simulink subsystem "RT_DynamicInflow_V1_2"  (R2025a)
settings: Solver=VariableStepAuto  StartTime=0.0  StopTime=100  RelTol=1e-3
model mask{RT_BEDistFromEffSta=0, RT_AirDensity=0, RT_RotorRadius=0}
  mask prompts: RT_BEDistFromEffSta "Blade element distance from effective station [-]"; RT_AirDensity "Air density [kgm^-3]"; RT_RotorRadius "Rotor radius [m]"
settings Model: DefaultTestHarness=RT_DynamicInflow_Harness1  Creator=Admin  LastModifiedBy=Admin

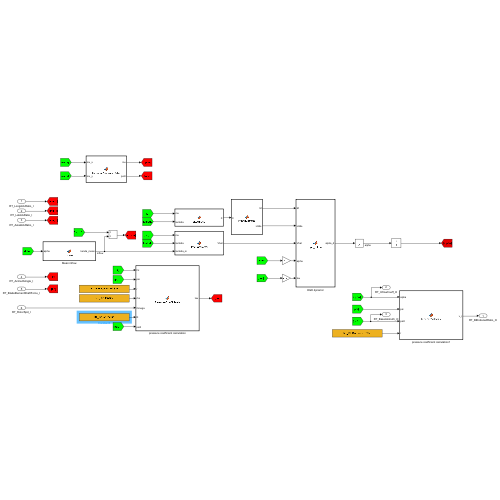
[thumbnail: Simulink's stored preview of the top-level diagram]
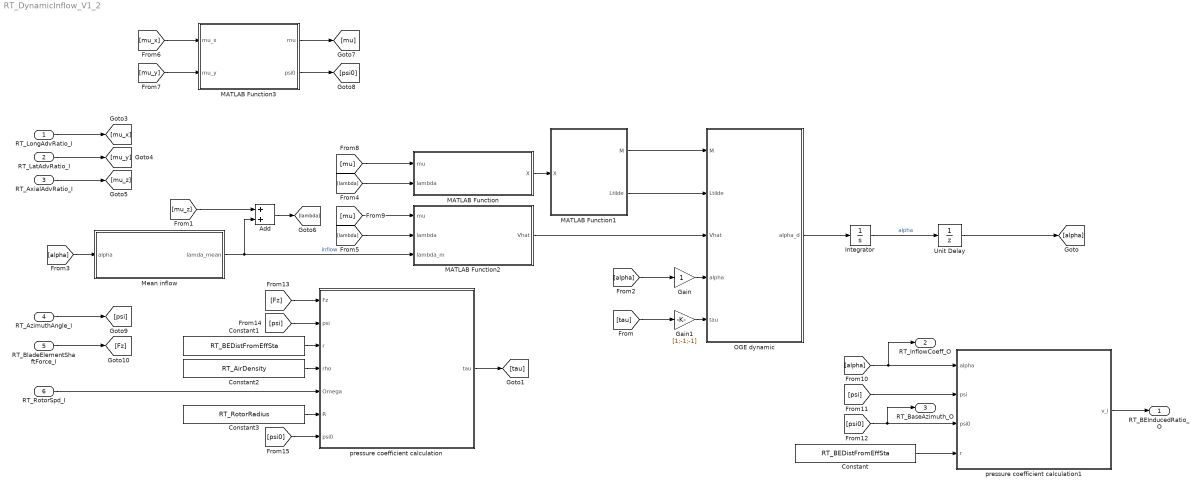
== system RT_DynamicInflow_V1_2 ==
  RT_LongAdvRatio_I : Inport
  RT_LatAdvRatio_I : Inport  Port=2
  RT_AxialAdvRatio_I : Inport  Port=3
  RT_AzimuthAngle_I : Inport  Port=4
  RT_BladeElementShaftForce_I : Inport  Port=5
  RT_RotorSpd_I : Inport  Port=6
  Add : Sum
  Constant : Constant  Value=RT_BEDistFromEffSta
  Constant1 : Constant  Value=RT_BEDistFromEffSta
  Constant2 : Constant  Value=RT_AirDensity
  Constant3 : Constant  Value=RT_RotorRadius
  Gain : Gain
  Gain1 : Gain  Gain=[1;-1;-1]
  Integrator : Integrator  InitialCondition=[0;0;0]
  MATLAB Function : MATLAB Function  TreatAsAtomicUnit=on
  MATLAB Function1 : MATLAB Function  TreatAsAtomicUnit=on
  MATLAB Function2 : MATLAB Function  TreatAsAtomicUnit=on
  MATLAB Function3 : MATLAB Function  TreatAsAtomicUnit=on
  Mean inflow : MATLAB Function  TreatAsAtomicUnit=on
  OGE dynamic : MATLAB Function  TreatAsAtomicUnit=on
  Unit Delay : UnitDelay  SampleTime=-1  HasFrameUpgradeWarning=on
  pressure coefficient calculation : MATLAB Function  TreatAsAtomicUnit=on
  pressure coefficient calculation1 : MATLAB Function  TreatAsAtomicUnit=on
  RT_BEInducedRatio_O : Outport
  RT_InflowCoeff_O : Outport  Port=2
  RT_BaseAzimuth_O : Outport  Port=3
  wires:
  MATLAB Function1/2(Ltilde) -> OGE dynamic/2(Ltilde)
  [alpha] -> Gain/1
  Unit Delay/1 -> [alpha]
  Mean inflow/1(lamda_mean) -> MATLAB Function2/3(lambda_m), Add/2  "inflow"
  Integrator/1 -> Unit Delay/1  "alpha"
  OGE dynamic/1(alpha_d) -> Integrator/1
  MATLAB Function/1(X) -> MATLAB Function1/1(X)
  MATLAB Function1/1(M) -> OGE dynamic/1(M)
  RT_LongAdvRatio_I/1 -> [mu_x]
  RT_LatAdvRatio_I/1 -> [mu_y]
  RT_AxialAdvRatio_I/1 -> [mu_z]
  [mu_z] -> Add/1
  Add/1 -> [lambda]
  [lambda] -> MATLAB Function/2(lambda)
  [lambda] -> MATLAB Function2/2(lambda)
  [mu_x] -> MATLAB Function3/1(mu_x)
  [mu_y] -> MATLAB Function3/2(mu_y)
  MATLAB Function3/1(mu) -> [mu]
  MATLAB Function3/2(psi0) -> [psi0]
  [mu] -> MATLAB Function/1(mu)
  [mu] -> MATLAB Function2/1(mu)
  [alpha] -> Mean inflow/1(alpha)
  [alpha] -> pressure coefficient calculation1/1(alpha), RT_InflowCoeff_O/1
  RT_AzimuthAngle_I/1 -> [psi]
  RT_BladeElementShaftForce_I/1 -> [Fz]
  [psi] -> pressure coefficient calculation1/2(psi)
  [psi0] -> pressure coefficient calculation1/3(psi0), RT_BaseAzimuth_O/1
  Constant/1 -> pressure coefficient calculation1/4(r)
  pressure coefficient calculation1/1(v_i) -> RT_BEInducedRatio_O/1
  Constant1/1 -> pressure coefficient calculation/3(r)
  Constant3/1 -> pressure coefficient calculation/6(R)
  Constant2/1 -> pressure coefficient calculation/4(rho)
  [Fz] -> pressure coefficient calculation/1(Fz)
  [psi] -> pressure coefficient calculation/2(psi)
  RT_RotorSpd_I/1 -> pressure coefficient calculation/5(Omega)
  pressure coefficient calculation/1(tau) -> [tau]
  [psi0] -> pressure coefficient calculation/7(psi0)
  MATLAB Function2/1(Vhat) -> OGE dynamic/3(Vhat)
  [tau] -> Gain1/1
  Gain/1 -> OGE dynamic/4(alpha)
  Gain1/1 -> OGE dynamic/5(tau)

== matlab function RT_DynamicInflow_V1_2/Mean inflow ==
  data: alpha input; lamda_mean output
function lamda_mean  = inflow(alpha)

lamda_mean = alpha(1)*sqrt(3);

== matlab function RT_DynamicInflow_V1_2/OGE dynamic ==
  data: M input; alpha_d output; Ltilde input; Vhat input; alpha input; tau input
function alpha_d = oge_inflow(M, Ltilde, Vhat, alpha, tau)
    alpha_d = M \ (0.5 * tau - (Ltilde \ (Vhat * alpha)));
end

== matlab function RT_DynamicInflow_V1_2/MATLAB Function ==
  data: mu input; X output; lambda input
function X = skewness(mu, lambda)
    VT = sqrt(mu^2 + lambda^2);

    if VT < 1e-6
        X = 0;
    else
        X = mu / (VT + abs(lambda));
    end
end

== matlab function RT_DynamicInflow_V1_2/MATLAB Function1 ==
  data: X input; M output; Ltilde output
function [M, Ltilde] = InflowMatrices(X)
    scale = [-1;-1;-1];
    M = diag([2/pi, -4/(3*pi), -4/(3*pi)]);
    
    % Ltilde = [ -1/4,          -X*pi/(2*sqrt(10)), 0; ...
    %             X*pi/sqrt(10), -(1-X^2)/24,       0; ...
    %             0,              0,                -(1+X^2)/24 ].*scale;
    Ltilde = [ 1/4,          X*pi/(2*sqrt(10)), 0; ...
            X*pi/sqrt(10), -(1-X^2)/24,       0; ...
            0,              0,                -(1+X^2)/24 ];
end

== matlab function RT_DynamicInflow_V1_2/pressure coefficient calculation ==
  data: Fz input; psi input; tau output; r input; rho input; Omega input; R input; psi0 input
function tau  = PressureCoefficients(Fz, psi, r, rho, Omega, R, psi0)
    [Nb, NSegment] = size(Fz);

    psi = psi(:)+psi0;          % Nb x 1
    r = r(:).';      % 1 x NSegment
    if numel(psi) ~= Nb
        error('Length of psi must equal number of blades (size(Fz,1)).');
    end
    if numel(r) ~= NSegment
        error('Length of rhat must equal number of segments (size(Fz,2)).');
    end

    % ---------- normalization ----------
    denom_m0 = 2 * pi * rho * Omega^2 * R^4; % Eq. 94
    denom_m1 =     pi * rho * Omega^2 * R^4; % Eqs. 92-93

    % ---------- shape functions ----------
    phi_01 = sqrt(3) * ones(1, NSegment);
    phi_12 = sqrt(15 / 2) * r;

    % ---------- azimuth factors ----------
    % One factor per blade, then expanded across segments
    c1 = cos(psi);   % Nb x 1
    s1 = sin(psi);   % Nb x 1

    % ---------- m = 0 cosine coefficients ----------
    % tau_n^{0c} = 1/(2*pi*rho*Omega^2*R^4) * sum_q sum_i L_i^q * phi_n^0(rhat_i)
    tau_01_c = sum(sum(Fz .* phi_01, 2), 1) / denom_m0;

    % ---------- m = 1 cosine/sine coefficients ----------
    % tau_n^{1c} = 1/(pi*rho*Omega^2*R^4) * sum_q sum_i L_i^q * phi_n^1(rhat_i) * cos(psi_q)
    % tau_n^{1s} = 1/(pi*rho*Omega^2*R^4) * sum_q sum_i L_i^q * phi_n^1(rhat_i) * sin(psi_q)

    % Expand azimuth factors over segments
    C = c1 * ones(1, NSegment);   % Nb x NSegment
    S = s1 * ones(1, NSegment);   % Nb x NSegment

    tau_12_c = sum(sum(Fz .* phi_12 .* C, 2), 1) / denom_m1;
    tau_12_s = sum(sum(Fz .* phi_12 .* S, 2), 1) / denom_m1;
    tau = [tau_01_c, tau_12_c, tau_12_s]';
    
end

== matlab function RT_DynamicInflow_V1_2/MATLAB Function2 ==
  data: mu input; Vhat output; lambda input; lambda_m input
function Vhat = FlowParameter(mu, lambda, lambda_m)
    VT = sqrt(mu^2 + lambda^2);

    if abs(VT) < 1e-6
        VT = 1e-6;
    end

    Vscalar = (mu^2 + (lambda + lambda_m) * lambda) / VT;
    Vhat    = diag([VT, Vscalar, Vscalar]);
end

== matlab function RT_DynamicInflow_V1_2/MATLAB Function3 ==
  data: mu_x input; mu output; psi0 output; mu_y input
function [mu,psi0] = ReorientAdvanceRatio(mu_x,mu_y)

psi0 = atan2(mu_y,mu_x);
if psi0 < 0
    psi0 = psi0+2*pi;
end
mu = sqrt(mu_x^2 + mu_y^2);

== matlab function RT_DynamicInflow_V1_2/pressure coefficient calculation1 ==
  data: alpha input; psi input; psi0 input; v_i output; r input
function v_i = InducedVelocity(alpha, psi, psi0, r)
% Nb not needed — already in solidity. Keep for compatibility but don't use.
v_i = sqrt(3)*alpha(1) + sqrt(15/2)*r'.*(alpha(2)*cos(psi+psi0)+alpha(3)*sin(psi+psi0));
end
